simulink model "aero_six_dof"  (R2019b)
settings: Solver=ode45  StartTime=0.0  StopTime=10  MaxStep=0.02  RelTol=1e-5  AbsTol=1e-7
undefined symbols (not defined in the file): pow
libraries: aerospace x7, simulink x6
Description:
  | Six Degrees of Freedom (6-DoF) Motion Platform
  | 
  | This example shows how to model six degrees of freedom motion in Simulink(R).
  | You can switch between using Euler Angles and Quaternions to model the
  | equations of motion, using the Variant Subsystem block's "Variant > Override using"
  | context menu.
settings Model: ExtModeTrigMode=oneshot  ExtModeArmWhenConnect=off  ExtModeAutoUpdateStatusClock=off  Creator=The MathWorks, Inc.  LastModifiedBy=Eduardo
settings SolverCC: AutoScaleAbsTol=off
settings DataIOCC: SaveFormat=Array  SaveOutput=off  ReturnWorkspaceOutputs=off  SignalLoggingName=sigsOut
settings OptimizationCC: BlockReduction=off  BooleanDataType=off  InitFltsAndDblsToZero=on  LifeSpan=inf
settings DebuggingCC: SaveWithParameterizedLinksMsg=none  SignalResolutionControl=TryResolveAllWithWarning  MultiTaskDSMMsg=warning  MultiTaskCondExecSysMsg=none  FcnCallInpInsideContextMsg=warning  SFUnexpectedBacktrackingDiag=warning  SFNoUnconditionalDefaultTransitionDiag=warning  SFExecutionAtInitializationDiag=none  ArithmeticOperatorsInVariantConditions=warning
settings HardwareCC: ProdBitPerPointer=32  ProdBitPerSizeT=32  ProdBitPerPtrDiffT=32  ProdLargestAtomicFloat=None  ProdIntDivRoundTo=Undefined  ProdEndianess=Unspecified  ProdWordSize=32  ProdHWDeviceType=32-bit Generic
settings ModelReferenceCC: PropagateSignalLabelsOutOfModel=off
settings SFSimCC: SimUseLocalCustomCode=off  CustomCodeUndefinedFunction=UseInterfaceOnly
settings RTWCC: TemplateMakefile=grt_vc.tmf  RTWUseLocalCustomCode=off
settings CodeAppCC: StateflowObjectComments=on
settings GRTTargetCC: TargetFcnLib=ansi_tfl_tmw.mat  TargetLangStandard=C89/C90 (ANSI)  GeneratePreprocessorConditionals=Disable all  CombineOutputUpdateFcns=off  GRTInterface=on
settings ConfigComp: CovMetricSettings=d  CovHtmlReporting=on  CovSaveCumulativeToWorkspaceVar=on  CovSaveSingleToWorkspaceVar=on  CovExternalEMLEnable=off  CovSFcnEnable=off

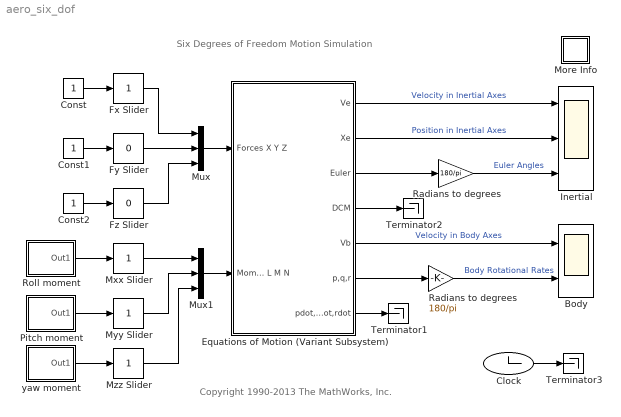
== system aero_six_dof ==
  note: Six Degrees of Freedom Motion Simulation
  note: Copyright 1990-2013 The MathWorks, Inc.
  Body : Scope  NumInputPorts=2
  Clock : Clock
      settings: Decimation=100
  Const : Constant
  Const1 : Constant
  Const2 : Constant
  Equations of Motion (Variant Subsystem) : Subsystem  VariantControlMode=Label  Variant=on  LabelModeActiveChoice=EqnMotion==1
  Fx Slider : simulink/Math Operations/Slider Gain  gain=1  low=-1  high=1
  Fy Slider : simulink/Math Operations/Slider Gain  gain=0  low=-1  high=1
  Fz Slider : simulink/Math Operations/Slider Gain  gain=0  low=-1  high=1
  Inertial : Scope  NumInputPorts=3
  More Info : Subsystem
      settings: OpenFcn=showdemo(bdroot(gcb))
      mask Display: disp('?')
  Mux : Mux  Inputs=3
  Mux1 : Mux  Inputs=3
  Mxx Slider : simulink/Math Operations/Slider Gain  gain=1  low=-5  high=10
  Myy Slider : simulink/Math Operations/Slider Gain  gain=1  low=-10  high=10
  Mzz Slider : simulink/Math Operations/Slider Gain  gain=1  low=-1  high=1
  Pitch moment : Subsystem  mask(timed input){t=[0 3 3 4 4 5 5  7.5 7.5 8.5 8.5 9.5 9.5 10], u=[0 0  1 1 -1 -1.005 0 0 -1 -1 1 1 0 0]*3.138/2}
      mask prompts: t "time values:"; u "input values"
      mask Display: plot(t,u)
  Radians to degrees : Gain  Gain=180/pi  SaturateOnIntegerOverflow=on  OutDataTypeStr=Inherit: Same as input  ParamDataTypeStr=Inherit: Same as input
  "Radians to degrees " : Gain  Gain=180/pi  SaturateOnIntegerOverflow=on  OutDataTypeStr=Inherit: Same as input  ParamDataTypeStr=Inherit: Same as input
  Roll moment : Subsystem  mask(timed input){t=[0 1 1 2 2  10], u=[1 1 -1 -.998  0 0]*3.144/2}
      mask prompts: t "time values:"; u "input values"
      mask Display: plot(t,u)
  Terminator1 : Terminator
  Terminator2 : Terminator
  Terminator3 : Terminator
  yaw moment : Subsystem  mask(timed input){t=[0 6 6 7 7 8 8 10], u=[0 0  -1 -1 1 1 0 0]*3.1/2}
      mask prompts: t "time values:"; u "input values"
      mask Display: plot(t,u)
  wires:
  yaw moment/1(Out1) -> Mzz Slider/1
  Pitch moment/1(Out1) -> Myy Slider/1
  Roll moment/1(Out1) -> Mxx Slider/1
  Const2/1 -> Fz Slider/1
  Const1/1 -> Fy Slider/1
  Const/1 -> Fx Slider/1
  Clock/1 -> Terminator3/1
  Mux1/1 -> Equations of Motion (Variant Subsystem)/2(Moments L M N)
  Mzz Slider/1 -> Mux1/3
  Myy Slider/1 -> Mux1/2
  Mxx Slider/1 -> Mux1/1
  Mux/1 -> Equations of Motion (Variant Subsystem)/1(Forces X Y Z)
  Fy Slider/1 -> Mux/2
  Fz Slider/1 -> Mux/3
  Fx Slider/1 -> Mux/1
  Equations of Motion (Variant Subsystem)/4(DCM) -> Terminator2/1
  Equations of Motion (Variant Subsystem)/7(pdot,qdot,rdot) -> Terminator1/1
  Equations of Motion (Variant Subsystem)/3(Euler) -> Radians to degrees/1
  Equations of Motion (Variant Subsystem)/5(Vb) -> Body/1  "Velocity in Body Axes"
  Equations of Motion (Variant Subsystem)/1(Ve) -> Inertial/1  "Velocity in Inertial Axes"
  Equations of Motion (Variant Subsystem)/2(Xe) -> Inertial/2  "Position in Inertial Axes"
  Radians to degrees/1 -> Inertial/3  "Euler Angles"
  Equations of Motion (Variant Subsystem)/6(p,q,r) -> "Radians to degrees "/1
  "Radians to degrees "/1 -> Body/2  "Body Rotational Rates"

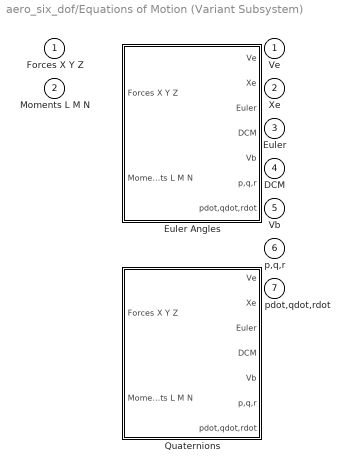
== system aero_six_dof/Equations of Motion (Variant Subsystem) ==
  Forces X Y Z : Inport
  Moments L M N : Inport  Port=2
  Euler Angles : Subsystem  VariantControl=EqnMotion==1  mask(6DoF Equations of Motion){xme_0=[0 0 0], Vm_0=[0 0 0], eul_0=[0 0 0], pm_0=[0 0 0], Mass=1.0, Inertia=eye(3)}
      mask prompts: xme_0 "Initial position in inertial axes [Xe,Ye,Ze]:"; Vm_0 "Initial velocity in body axes [U,v,w]:"; eul_0 "Initial Euler orientation [roll, pitch, yaw]:"; pm_0 "Initial body rotation rates [p,q,r]:"; Inertia "Inertia matrix:"
      mask help: Integrates the 6 degrees of freedom equations of motion using an euler angle representation for the orientation of the body in space.
      mask Help:
      | <p>This block models a 6 degrees of freedom equations of motion for a rigid body using an euler angle representation.</p>
      | 
      | <pThe block inputs and outputs contain more than one signal as described below.</p>
      | 
      | <p><H4>Block Vector  Input - Forces X Y Z</H4>
      | <ul>
      |     <li>Forces on the body in X direction - X </li>
      |     <li>Forces on the body in Y direction - Y </li>
      |     <li>Forces on the body in Z direction - Z </li>
      | </ul>
      | </p>
      | <p><H4>Block Vector  Input - Moments L M N</H4>
      | <ul>
      |     <li>Moments on the body along X direction - L </li>
      |     <li>Moments on the body along Y direction - M </li>
      |     <li>Moments on the body along Z direction - N </li>
      | </ul>
      | </p>
      | <p><H4>Block Vector Output - Ve </H4>
      | <ul>
      |     <li>Translational velocity in X direction in Inertial coordinates </li>
      |     <li>Translational velocity in Y direction in Inertial coordinates </li>
      |     <li>Translational velocity in Z direction in Inertial coordinates </li>
      | </ul>
      | </p>
      | <p><H4>Block Vector Output - Xe </H4>
      | <ul>
      |     <li>Position in X direction in Inertial coordinates - Xe </li>
      |     <li>Position in Y direction in Inertial coordinates - Ye </li>
      |     <li>Position in Z direction in Inertial coordinates - Ze </li>
      | </ul>
      | </p>
      | <p><H4>Block Vector Output - Euler </H4>
      | <ul>
      |     <li>Phi ( radians )</li>
      |     <li>Theta ( radians )</li>
      |     <li>Psi ( radians )</li>
      | </ul>
      | </p>
      | <p><H4>Block Vector Output - DMC </H4>
      | <ul>
      |     <li>3x3 Directional Cosine Matrix</li>
      | </ul>
      | </p>
      | <p><H4>Block Vector Output - Vb</H4>
      | <ul>
      |     <li>Translational velocity in X direction in Body coordinates </li>
      |     <li>Translational velocity in Y direction in Body coordinates </li>
      |     <li>Translational velocity in Z direction in Body coordinates </li>
      | </ul>
      | </p>
      | <p><H4>Block Vector Output - p, q, r</H4>
      | <ul>
      |     <li>Roll rate - p ( radians/sec )</li>
      |     <li>Pitch rate - q ( radians/sec )</li>
      |     <li>Yaw rate - r ( radians/sec )</li>
      | </ul>
      | </p>
      | <p><H4>Block Vector Output - pdot, qdot, rdot</H4>
      | <ul>
      |     <li>Roll acceleration - pdot ( radians/sec^2 )</li>
      |     <li>Pitch acceleration - qdot ( radians/sec^2 )</li>
      |     <li>Yaw acceleration - rdot ( radians/sec^2 )</li>
      | </ul>
      | </p>
      mask Display: disp('Euler\nAngles')
  Quaternions : Subsystem  VariantControl=EqnMotion==2  mask(6DoF Equations of Motion){xme_0=[0 0 0], Vm_0=[0 0 0], eul_0=[0 0 0], pm_0=[0 0 0], Mass=1.0, Inertia=eye(3)}
      mask prompts: xme_0 "Initial position in inertial axes [Xe,Ye,Ze]:"; Vm_0 "Initial velocity in body axes [U,v,w]:"; eul_0 "Initial Euler orientation [roll, pitch, yaw]:"; pm_0 "Initial body rotation rates [p,q,r]:"; Inertia "Inertia matrix:"
      mask help: Integrates the 6 degrees of freedom equations of motion using a quaternion representation for the orientation of the body in space.
      mask init:
      | %%% factor used for quaternion calculation
      | k_quat=100;
      | 
      | %%% initial orientation of platform
      | ph=eul_0(1);
      | th=eul_0(2);
      | ps=eul_0(3);
      | e0_0 = cos(0.5*ps)*cos(0.5*th)*cos(0.5*ph) +sin(0.5*ps)*sin(0.5*th)*sin(0.5*ph);
      | e1_0 = cos(0.5*ps)*cos(0.5*th)*sin(0.5*ph) - sin(0.5*ps)*sin(0.5*th)*cos(0.5*ph);
      | e2_0 = cos(0.5*ps)*sin(0.5*th)*cos(0.5*ph) +sin(0.5*ps)*cos(0.5*th)*sin(0.5*ph);
      | e3_0 =-cos(0.5*ps)*sin(0.5*th)*sin(0.5*ph) +sin(0.5*ps)*cos(0.5*th)*cos(0.5*ph);
      mask Help:
      | <p>This block models a 6 degrees of freedom equations of motion for a rigid body using a quaternion representation.</p>
      | 
      | <pThe block inputs and outputs contain more than one signal as described below.</p>
      | 
      | <p><H4>Block Vector  Input - Forces X Y Z</H4>
      | <ul>
      |     <li>Forces on the body in X direction - X </li>
      |     <li>Forces on the body in Y direction - Y </li>
      |     <li>Forces on the body in Z direction - Z </li>
      | </ul>
      | </p>
      | <p><H4>Block Vector  Input - Moments L M N</H4>
      | <ul>
      |     <li>Moments on the body along X direction - L </li>
      |     <li>Moments on the body along Y direction - M </li>
      |     <li>Moments on the body along Z direction - N </li>
      | </ul>
      | </p>
      | <p><H4>Block Vector Output - Ve </H4>
      | <ul>
      |     <li>Translational velocity in X direction in Inertial coordinates </li>
      |     <li>Translational velocity in Y direction in Inertial coordinates </li>
      |     <li>Translational velocity in Z direction in Inertial coordinates </li>
      | </ul>
      | </p>
      | <p><H4>Block Vector Output - Xe </H4>
      | <ul>
      |     <li>Position in X direction in Inertial coordinates - Xe </li>
      |     <li>Position in Y direction in Inertial coordinates - Ye </li>
      |     <li>Position in Z direction in Inertial coordinates - Ze </li>
      | </ul>
      | </p>
      | <p><H4>Block Vector Output - Euler </H4>
      | <ul>
      |     <li>Phi ( radians )</li>
      |     <li>Theta ( radians )</li>
      |     <li>Psi ( radians )</li>
      | </ul>
      | </p>
      | <p><H4>Block Vector Output - DMC </H4>
      | <ul>
      |     <li>3x3 Directional Cosine Matrix</li>
      | </ul>
      | </p>
      | <p><H4>Block Vector Output - Vb</H4>
      | <ul>
      |     <li>Translational velocity in X direction in Body coordinates </li>
      |     <li>Translational velocity in Y direction in Body coordinates </li>
      |     <li>Translational velocity in Z direction in Body coordinates </li>
      | </ul>
      | </p>
      | <p><H4>Block Vector Output - p, q, r</H4>
      | <ul>
      |     <li>Roll rate - p ( radians/sec )</li>
      |     <li>Pitch rate - q ( radians/sec )</li>
      |     <li>Yaw rate - r ( radians/sec )</li>
      | </ul>
      | </p>
      | <p><H4>Block Vector Output - pdot, qdot, rdot</H4>
      | <ul>
      |     <li>Roll acceleration - pdot ( radians/sec^2 )</li>
      |     <li>Pitch acceleration - qdot ( radians/sec^2 )</li>
      |     <li>Yaw acceleration - rdot ( radians/sec^2 )</li>
      | </ul>
      | </p>
      mask Display: disp('Quaternions')
  Ve : Outport  VectorParamsAs1DForOutWhenUnconnected=off
  Xe : Outport  Port=2  VectorParamsAs1DForOutWhenUnconnected=off
  Euler : Outport  Port=3  VectorParamsAs1DForOutWhenUnconnected=off
  DCM : Outport  Port=4  VectorParamsAs1DForOutWhenUnconnected=off
  Vb : Outport  Port=5  VectorParamsAs1DForOutWhenUnconnected=off
  p,q,r : Outport  Port=6  VectorParamsAs1DForOutWhenUnconnected=off
  pdot,qdot,rdot : Outport  Port=7  VectorParamsAs1DForOutWhenUnconnected=off

== system aero_six_dof/More Info ==

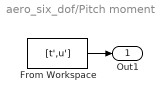
== system aero_six_dof/Pitch moment ==
  From Workspace : FromWorkspace  VariableName=[t',u']  SampleTime=0
  Out1 : Outport  InitialOutput=0  VectorParamsAs1DForOutWhenUnconnected=off
  wires:
  From Workspace/1 -> Out1/1

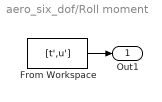
== system aero_six_dof/Roll moment ==
  From Workspace : FromWorkspace  VariableName=[t',u']  SampleTime=0
  Out1 : Outport  InitialOutput=0  VectorParamsAs1DForOutWhenUnconnected=off
  wires:
  From Workspace/1 -> Out1/1

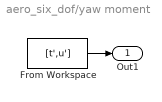
== system aero_six_dof/yaw moment ==
  From Workspace : FromWorkspace  VariableName=[t',u']  SampleTime=0
  Out1 : Outport  InitialOutput=0  VectorParamsAs1DForOutWhenUnconnected=off
  wires:
  From Workspace/1 -> Out1/1

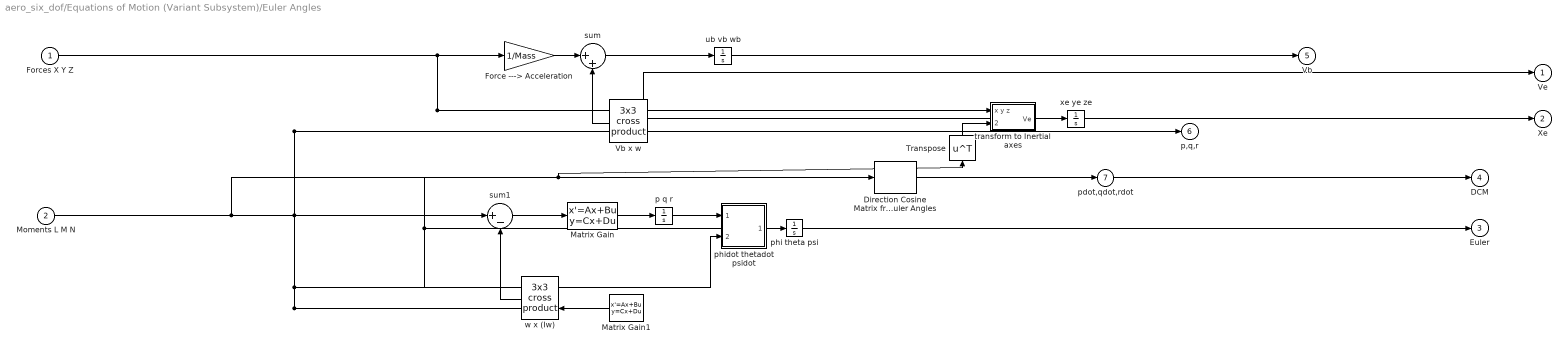
== system aero_six_dof/Equations of Motion (Variant Subsystem)/Euler Angles ==
  Forces X Y Z : Inport
  Moments L M N : Inport  Port=2
  Direction Cosine Matrix from Euler Angles : aerospace/Axes Transformations/Direction Cosine Matrix from Euler Angles
  Force ---> Acceleration : Gain  Gain=1/Mass  SaturateOnIntegerOverflow=on  OutDataTypeStr=Inherit: Same as input  ParamDataTypeStr=Inherit: Same as input
  Matrix Gain : StateSpace  A=[]  B=[]  C=[]  D=K  InitialCondition=0  mask(Matrix Gain){K=inv(Inertia)}
      mask prompts: K "Gain matrix:"
      mask help: Matrix Gain.
      mask Help: Multiplies input vector by entered matrix to produce output vector (y=Au).
      mask Display: disp('Inertia^(-1)')
  Matrix Gain1 : StateSpace  A=[]  B=[]  C=[]  D=K  InitialCondition=0  mask(Matrix Gain){K=Inertia}
      mask prompts: K "Gain matrix:"
      mask help: Matrix Gain.
      mask Help: Multiplies input vector by entered matrix to produce output vector (y=Au).
      mask Display: disp('Inertia')
  Transpose : Math  Operator=transpose  SaturateOnIntegerOverflow=on
  Vb x w : aerospace/Axes Transformations/3x3 cross product
  p q r : Integrator  InitialCondition=pm_0
  phi theta psi : Integrator  InitialCondition=eul_0
  phidot thetadot psidot : Subsystem
  sum : Sum  Inputs=|++  SaturateOnIntegerOverflow=on  InputSameDT=on  OutDataTypeStr=Inherit: Same as first input
  sum1 : Sum  Inputs=|+-  SaturateOnIntegerOverflow=on  InputSameDT=on  OutDataTypeStr=Inherit: Same as first input
  "transform to Inertial axes " : Subsystem  mask(Vector Transformation){}
      mask Display: disp('L_EB')
  ub vb wb : Integrator  InitialCondition=Vm_0
  w x (Iw) : aerospace/Axes Transformations/3x3 cross product
  xe ye ze : Integrator  InitialCondition=xme_0
  Ve : Outport  InitialOutput=0  VectorParamsAs1DForOutWhenUnconnected=off
  Xe : Outport  Port=2  InitialOutput=0  VectorParamsAs1DForOutWhenUnconnected=off
  Euler : Outport  Port=3  InitialOutput=0  VectorParamsAs1DForOutWhenUnconnected=off
  DCM : Outport  Port=4  InitialOutput=0  VectorParamsAs1DForOutWhenUnconnected=off
  Vb : Outport  Port=5  InitialOutput=0  VectorParamsAs1DForOutWhenUnconnected=off
  p,q,r : Outport  Port=6  InitialOutput=0  VectorParamsAs1DForOutWhenUnconnected=off
  pdot,qdot,rdot : Outport  Port=7  InitialOutput=0  VectorParamsAs1DForOutWhenUnconnected=off
  wires:
  phidot thetadot psidot/1(phidot thetadot psi) -> phi theta psi/1
  phi theta psi/1 -> Euler/1, phidot thetadot psidot/2(phi theta psi), Direction Cosine Matrix from Euler Angles/1
  ub vb wb/1 -> Vb/1, Vb x w/1, "transform to Inertial axes "/1(x y z)
  sum/1 -> ub vb wb/1
  xe ye ze/1 -> Xe/1
  "transform to Inertial axes "/1(Ve) -> xe ye ze/1, Ve/1
  p q r/1 -> Vb x w/2, p,q,r/1, Matrix Gain1/1, phidot thetadot psidot/1(p q r), w x (Iw)/1
  sum1/1 -> Matrix Gain/1
  Moments L M N/1 -> sum1/1
  Matrix Gain1/1 -> w x (Iw)/2
  w x (Iw)/1 -> sum1/2
  Matrix Gain/1 -> p q r/1, pdot,qdot,rdot/1
  Forces X Y Z/1 -> Force ---> Acceleration/1
  Vb x w/1 -> sum/2
  Force ---> Acceleration/1 -> sum/1
  Direction Cosine Matrix from Euler Angles/1 -> Transpose/1, DCM/1
  Transpose/1 -> "transform to Inertial axes "/2(transform coefficients)

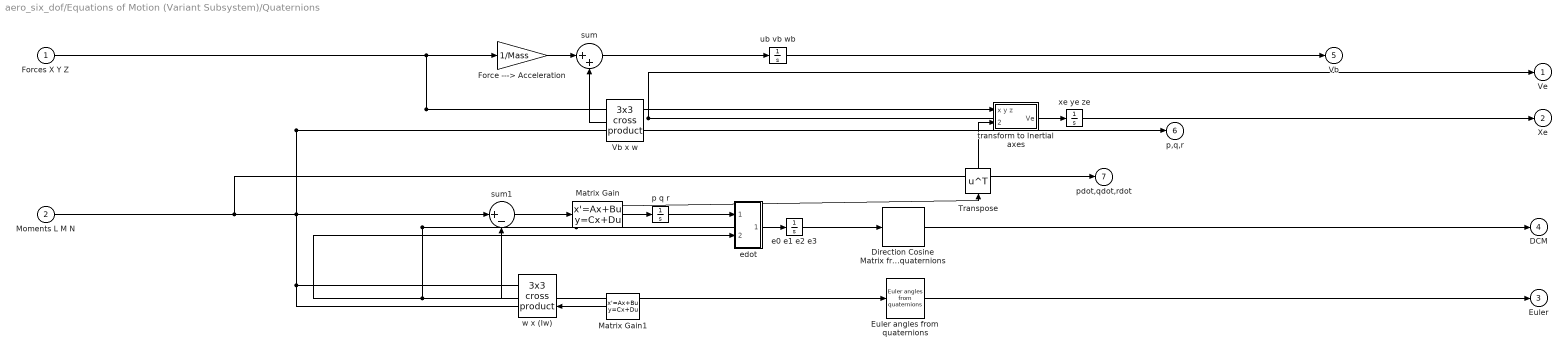
== system aero_six_dof/Equations of Motion (Variant Subsystem)/Quaternions ==
  Forces X Y Z : Inport
  Moments L M N : Inport  Port=2
  Direction Cosine Matrix from quaternions : aerospace/Axes Transformations/Direction Cosine Matrix from quaternions
  Euler angles from quaternions : aerospace/Axes Transformations/Euler angles from quaternions
  Force ---> Acceleration : Gain  Gain=1/Mass  SaturateOnIntegerOverflow=on  OutDataTypeStr=Inherit: Same as input  ParamDataTypeStr=Inherit: Same as input
  Matrix Gain : StateSpace  A=[]  B=[]  C=[]  D=K  InitialCondition=0  mask(Matrix Gain){K=inv(Inertia)}
      mask prompts: K "Gain matrix:"
      mask help: Matrix Gain.
      mask Help: Multiplies input vector by entered matrix to produce output vector (y=Au).
      mask Display: disp('Inertia^(-1)')
  Matrix Gain1 : StateSpace  A=[]  B=[]  C=[]  D=K  InitialCondition=0  mask(Matrix Gain){K=Inertia}
      mask prompts: K "Gain matrix:"
      mask help: Matrix Gain.
      mask Help: Multiplies input vector by entered matrix to produce output vector (y=Au).
      mask Display: disp('Inertia')
  Transpose : Math  Operator=transpose  SaturateOnIntegerOverflow=on
  Vb x w : aerospace/Axes Transformations/3x3 cross product
  e0 e1 e2 e3 : Integrator  InitialCondition=[e0_0 e1_0 e2_0 e3_0]
  edot : Subsystem
  p q r : Integrator  InitialCondition=pm_0
  sum : Sum  Inputs=|++  SaturateOnIntegerOverflow=on  InputSameDT=on  OutDataTypeStr=Inherit: Same as first input
  sum1 : Sum  Inputs=|+-  SaturateOnIntegerOverflow=on  InputSameDT=on  OutDataTypeStr=Inherit: Same as first input
  "transform to Inertial axes " : Subsystem  mask(Vector Transformation){}
      mask Display: disp('L_EB')
  ub vb wb : Integrator  InitialCondition=Vm_0
  w x (Iw) : aerospace/Axes Transformations/3x3 cross product
  xe ye ze : Integrator  InitialCondition=xme_0
  Ve : Outport  InitialOutput=0  VectorParamsAs1DForOutWhenUnconnected=off
  Xe : Outport  Port=2  InitialOutput=0  VectorParamsAs1DForOutWhenUnconnected=off
  Euler : Outport  Port=3  InitialOutput=0  VectorParamsAs1DForOutWhenUnconnected=off
  DCM : Outport  Port=4  InitialOutput=0  VectorParamsAs1DForOutWhenUnconnected=off
  Vb : Outport  Port=5  InitialOutput=0  VectorParamsAs1DForOutWhenUnconnected=off
  p,q,r : Outport  Port=6  InitialOutput=0  VectorParamsAs1DForOutWhenUnconnected=off
  pdot,qdot,rdot : Outport  Port=7  InitialOutput=0  VectorParamsAs1DForOutWhenUnconnected=off
  wires:
  p q r/1 -> edot/1(in_1), Vb x w/2, p,q,r/1, Matrix Gain1/1, w x (Iw)/1
  sum1/1 -> Matrix Gain/1
  Moments L M N/1 -> sum1/1
  Matrix Gain1/1 -> w x (Iw)/2
  w x (Iw)/1 -> sum1/2
  edot/1(out_1) -> e0 e1 e2 e3/1
  e0 e1 e2 e3/1 -> Direction Cosine Matrix from quaternions/1, Euler angles from quaternions/1, edot/2(in_2)
  Euler angles from quaternions/1 -> Euler/1
  Matrix Gain/1 -> p q r/1, pdot,qdot,rdot/1
  Direction Cosine Matrix from quaternions/1 -> Transpose/1, DCM/1
  ub vb wb/1 -> Vb/1, Vb x w/1, "transform to Inertial axes "/1(x y z)
  Forces X Y Z/1 -> Force ---> Acceleration/1
  Vb x w/1 -> sum/2
  sum/1 -> ub vb wb/1
  Force ---> Acceleration/1 -> sum/1
  xe ye ze/1 -> Xe/1
  "transform to Inertial axes "/1(Ve) -> xe ye ze/1, Ve/1
  Transpose/1 -> "transform to Inertial axes "/2(transform coefficients)

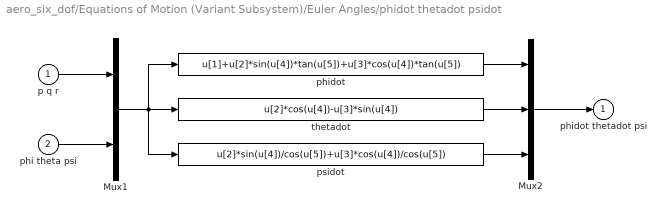
== system aero_six_dof/Equations of Motion (Variant Subsystem)/Euler Angles/phidot thetadot psidot ==
  p q r : Inport
  phi theta psi : Inport  Port=2
  Mux1 : Mux  Inputs=[3 3]
  Mux2 : Mux  Inputs=3
  phidot : Fcn  Expr=u[1]+u[2]*sin(u[4])*tan(u[5])+u[3]*cos(u[4])*tan(u[5])
  psidot : Fcn  Expr=u[2]*sin(u[4])/cos(u[5])+u[3]*cos(u[4])/cos(u[5])
  thetadot : Fcn  Expr=u[2]*cos(u[4])-u[3]*sin(u[4])
  phidot thetadot psi : Outport  InitialOutput=0  VectorParamsAs1DForOutWhenUnconnected=off
  wires:
  Mux1/1 -> psidot/1, phidot/1, thetadot/1
  p q r/1 -> Mux1/1
  phi theta psi/1 -> Mux1/2
  psidot/1 -> Mux2/3
  thetadot/1 -> Mux2/2
  phidot/1 -> Mux2/1
  Mux2/1 -> phidot thetadot psi/1

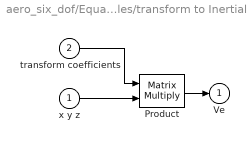
== system aero_six_dof/Equations of Motion (Variant Subsystem)/Euler Angles/transform to Inertial axes  ==
  x y z : Inport
  transform coefficients : Inport  Port=2
  Product : Product  Multiplication=Matrix(*)  SaturateOnIntegerOverflow=on  RndMeth=Zero  InputSameDT=on  OutDataTypeStr=Inherit: Same as first input
  Ve : Outport  InitialOutput=0  VectorParamsAs1DForOutWhenUnconnected=off
  wires:
  x y z/1 -> Product/2
  transform coefficients/1 -> Product/1
  Product/1 -> Ve/1

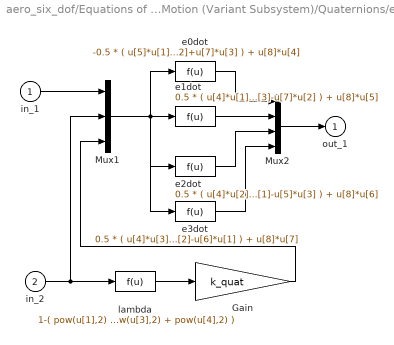
== system aero_six_dof/Equations of Motion (Variant Subsystem)/Quaternions/edot ==
  in_1 : Inport
  in_2 : Inport  Port=2
  Gain : Gain  Gain=k_quat  SaturateOnIntegerOverflow=on  OutDataTypeStr=Inherit: Same as input  ParamDataTypeStr=Inherit: Same as input
  Mux1 : Mux  Inputs=[3 4 1]
  Mux2 : Mux
  e0dot : Fcn  Expr=-0.5 * ( u[5]*u[1]+u[6]*u[2]+u[7]*u[3] ) + u[8]*u[4]
  e1dot : Fcn  Expr=0.5 * ( u[4]*u[1]+u[6]*u[3]-u[7]*u[2] ) + u[8]*u[5]
  e2dot : Fcn  Expr=0.5 * ( u[4]*u[2]+u[7]*u[1]-u[5]*u[3] ) + u[8]*u[6]
  e3dot : Fcn  Expr=0.5 * ( u[4]*u[3]+u[5]*u[2]-u[6]*u[1] ) + u[8]*u[7]
  lambda : Fcn  Expr=1-( pow(u[1],2) + pow(u[2],2) + pow(u[3],2) + pow(u[4],2) )
  out_1 : Outport  InitialOutput=0  VectorParamsAs1DForOutWhenUnconnected=off
  wires:
  Mux2/1 -> out_1/1
  in_1/1 -> Mux1/1
  e0dot/1 -> Mux2/1
  e1dot/1 -> Mux2/2
  e2dot/1 -> Mux2/3
  Mux1/1 -> e0dot/1, e1dot/1, e2dot/1, e3dot/1
  e3dot/1 -> Mux2/4
  lambda/1 -> Gain/1
  Gain/1 -> Mux1/3
  in_2/1 -> lambda/1, Mux1/2

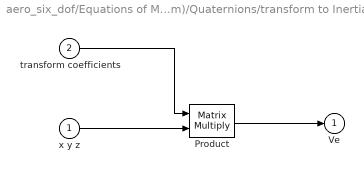
== system aero_six_dof/Equations of Motion (Variant Subsystem)/Quaternions/transform to Inertial axes  ==
  x y z : Inport
  transform coefficients : Inport  Port=2
  Product : Product  Multiplication=Matrix(*)  SaturateOnIntegerOverflow=on  RndMeth=Zero  InputSameDT=on  OutDataTypeStr=Inherit: Same as first input
  Ve : Outport  InitialOutput=0  VectorParamsAs1DForOutWhenUnconnected=off
  wires:
  Product/1 -> Ve/1
  transform coefficients/1 -> Product/1
  x y z/1 -> Product/2
